simulink library "satelliteDynamics_lib_2"  (R2018b)
settings: Solver=VariableStepAuto  StartTime=0.0  StopTime=10.0  RelTol=1e-3
undefined symbols (not defined in the file or in its folder): DiscIntNeverNeededParam, fswParams, simParams
libraries: vrlib x1, aerolibutil x1, sharedutil x1
settings Model: Creator=colem  LastModifiedBy=colem

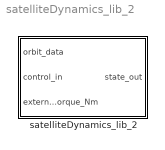
== system satelliteDynamics_lib_2 ==
  satelliteDynamics_lib_2 : Subsystem

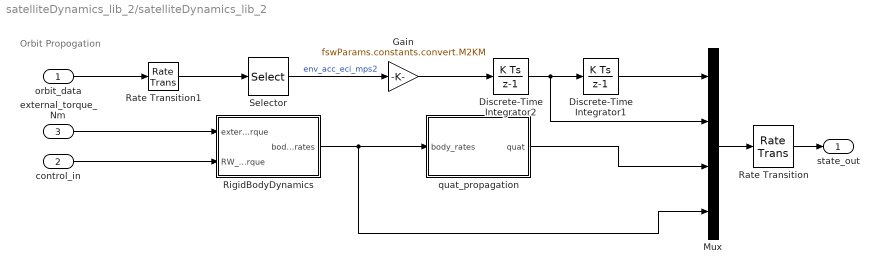
== system satelliteDynamics_lib_2/satelliteDynamics_lib_2 ==
  note: Orbit Propogation
  orbit_data : Inport
  control_in : Inport  Port=2
  external_torque_Nm : Inport  Port=3
  Discrete-Time Integrator1 : DiscreteIntegrator  InitialCondition=simParams.initialConditions.r0  SampleTime=-1  ICPrevOutput=DiscIntNeverNeededParam  ICPrevScaledInput=DiscIntNeverNeededParam
  Discrete-Time Integrator2 : DiscreteIntegrator  InitialCondition=simParams.initialConditions.v0  SampleTime=-1  ICPrevOutput=DiscIntNeverNeededParam  ICPrevScaledInput=DiscIntNeverNeededParam
  Gain : Gain  Gain=fswParams.constants.convert.M2KM
  Mux : Mux  Inputs=[3 3 4 3]
  Rate Transition : RateTransition  InitialCondition=[simParams.initialConditions.r0;simParams.initialConditions.v0;simParams.initialConditions.q0;simParams.initialConditions.w0]
  Rate Transition1 : RateTransition  OutPortSampleTime=simParams.sample_time_s
  RigidBodyDynamics : Subsystem
  Selector : Selector  InputPortWidth=13  IndexOptions=Index vector (dialog)  Indices=[1 2 3]  OutputSizes=1
  quat_propagation : Subsystem
  state_out : Outport
  wires:
  control_in/1 -> RigidBodyDynamics/2(RW_torque)
  Mux/1 -> Rate Transition/1
  Discrete-Time Integrator2/1 -> Discrete-Time Integrator1/1, Mux/2
  Discrete-Time Integrator1/1 -> Mux/1
  Gain/1 -> Discrete-Time Integrator2/1
  Rate Transition/1 -> state_out/1
  orbit_data/1 -> Rate Transition1/1
  Rate Transition1/1 -> Selector/1
  external_torque_Nm/1 -> RigidBodyDynamics/1(external_torque)
  Selector/1 -> Gain/1  "env_acc_eci_mps2"
  quat_propagation/1(quat) -> Mux/3
  RigidBodyDynamics/1(body_rates) -> Mux/4, quat_propagation/1(body_rates)

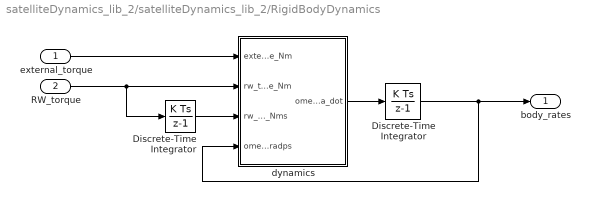
== system satelliteDynamics_lib_2/satelliteDynamics_lib_2/RigidBodyDynamics ==
  external_torque : Inport
  RW_torque : Inport  Port=2
  Discrete-Time Integrator : DiscreteIntegrator  InitialCondition=[0;0;0]  SampleTime=-1  ICPrevOutput=DiscIntNeverNeededParam  ICPrevScaledInput=DiscIntNeverNeededParam
  "Discrete-Time Integrator " : DiscreteIntegrator  InitialCondition=simParams.initialConditions.w0  SampleTime=-1  ICPrevOutput=DiscIntNeverNeededParam  ICPrevScaledInput=DiscIntNeverNeededParam
  dynamics : Subsystem
  body_rates : Outport
  wires:
  RW_torque/1 -> dynamics/2(rw_torque_Nm), Discrete-Time Integrator/1
  Discrete-Time Integrator/1 -> dynamics/3(rw_momentum_Nms)
  "Discrete-Time Integrator "/1 -> body_rates/1, dynamics/4(omega_radps)
  external_torque/1 -> dynamics/1(external_torque_Nm)
  dynamics/1(omega_dot) -> "Discrete-Time Integrator "/1

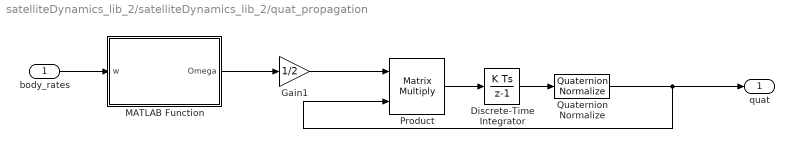
== system satelliteDynamics_lib_2/satelliteDynamics_lib_2/quat_propagation ==
  body_rates : Inport
  Discrete-Time Integrator : DiscreteIntegrator  InitialCondition=simParams.initialConditions.q0  SampleTime=-1  ICPrevOutput=DiscIntNeverNeededParam  ICPrevScaledInput=DiscIntNeverNeededParam
  Gain1 : Gain  Gain=1/2
  MATLAB Function : MATLAB Function  TreatAsAtomicUnit=on
  Product : Product  Multiplication=Matrix(*)  RndMeth=Zero
  Quaternion Normalize : sharedutil/Quaternion Normalize  aMode=aMode
      settings: SourceProductName=Aerospace Blockset  SourceProductBaseCode=AE
  quat : Outport
  wires:
  Product/1 -> Discrete-Time Integrator/1
  Discrete-Time Integrator/1 -> Quaternion Normalize/1
  Gain1/1 -> Product/1
  Quaternion Normalize/1 -> quat/1, Product/2
  body_rates/1 -> MATLAB Function/1(w)
  MATLAB Function/1(Omega) -> Gain1/1

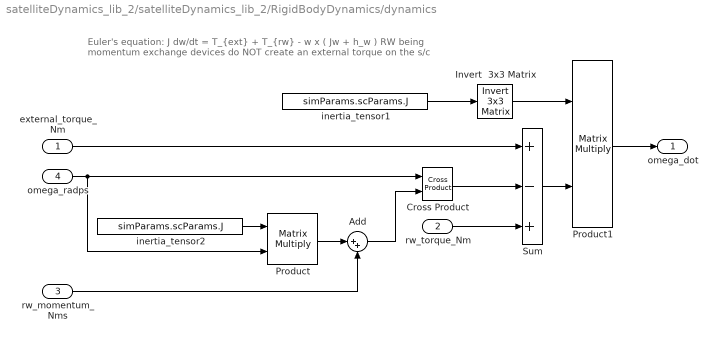
== system satelliteDynamics_lib_2/satelliteDynamics_lib_2/RigidBodyDynamics/dynamics ==
  note: Euler's equation: J dw/dt = T_{ext} + T_{rw} - w x ( Jw + h_w )
      |
      | RW being momentum exchange devices do NOT create
      | an external torque on the s/c
  external_torque_Nm : Inport
  rw_torque_Nm : Inport  Port=2
  rw_momentum_Nms : Inport  Port=3
  omega_radps : Inport  Port=4
  Add : Sum  Inputs=|++
  Cross Product : vrlib/Utilities/Cross Product
      settings: SourceProductBaseCode=VR
  Invert  3x3 Matrix : aerolibutil/Invert  3x3 Matrix
  Product : Product  Multiplication=Matrix(*)  RndMeth=Zero
  Product1 : Product  Multiplication=Matrix(*)  RndMeth=Zero
  Sum : Sum  Inputs=+-+
  inertia_tensor1 : Constant  Value=simParams.scParams.J  SampleTime=simParams.sample_time_s
  inertia_tensor2 : Constant  Value=simParams.scParams.J  SampleTime=simParams.sample_time_s
  omega_dot : Outport
  wires:
  rw_torque_Nm/1 -> Sum/3
  Add/1 -> Cross Product/2
  Product/1 -> Add/1
  Cross Product/1 -> Sum/2
  inertia_tensor1/1 -> Invert  3x3 Matrix/1
  Invert  3x3 Matrix/1 -> Product1/1
  Product1/1 -> omega_dot/1
  Sum/1 -> Product1/2
  inertia_tensor2/1 -> Product/1
  omega_radps/1 -> Cross Product/1, Product/2
  external_torque_Nm/1 -> Sum/1
  rw_momentum_Nms/1 -> Add/2

== matlab function satelliteDynamics_lib_2/quat_propagation/MATLAB Function ==
  data: w input; Omega output
function Omega = skew_sym(w)
%#codegen

    w_skew = ...
        [0 w(3) -w(2);
        -w(3) 0 w(1);
        w(2) -w(1) 0];

    Omega = ...
        [0 -w';
        w w_skew];
